simulink model "linear_feedback"  (R2021b)
settings: Solver=VariableStepAuto  StartTime=0.0  StopTime=10.0  RelTol=1e-3
undefined symbols (not defined in the file): magnitude
settings Model: Creator=84232  LastModifiedBy=84232

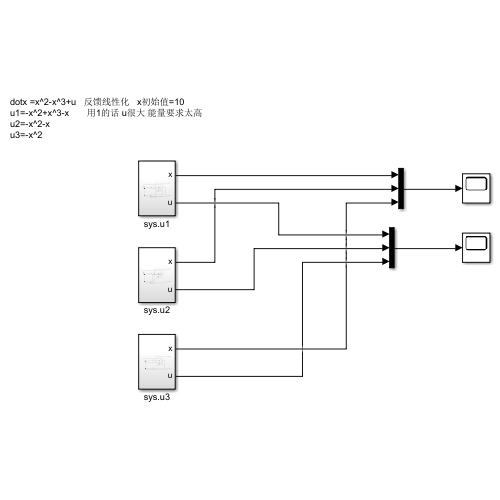
[thumbnail: Simulink's stored preview of the top-level diagram]
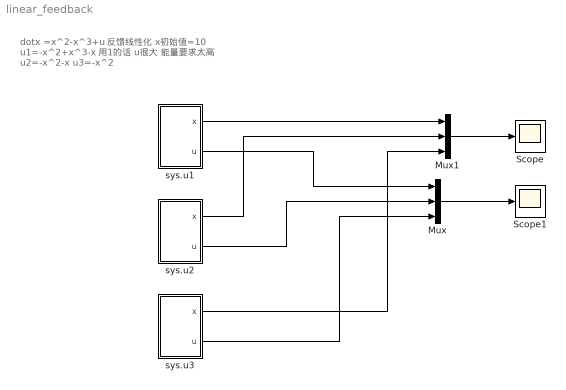
== system linear_feedback ==
  note: dotx =x^2-x^3+u   反馈线性化   x初始值=10
      | u1=-x^2+x^3-x       用1的话 u很大 能量要求太高
      | u2=-x^2-x
      | u3=-x^2
  Mux : Mux  Inputs=3
  Mux1 : Mux  Inputs=3
  Scope : Scope
  Scope1 : Scope
  sys.u1 : Subsystem
  sys.u2 : Subsystem
  sys.u3 : Subsystem
  wires:
  sys.u1/2(u) -> Mux/1
  sys.u2/2(u) -> Mux/2
  sys.u3/2(u) -> Mux/3
  Mux/1 -> Scope1/1
  sys.u1/1(x) -> Mux1/1
  sys.u2/1(x) -> Mux1/2
  sys.u3/1(x) -> Mux1/3
  Mux1/1 -> Scope/1

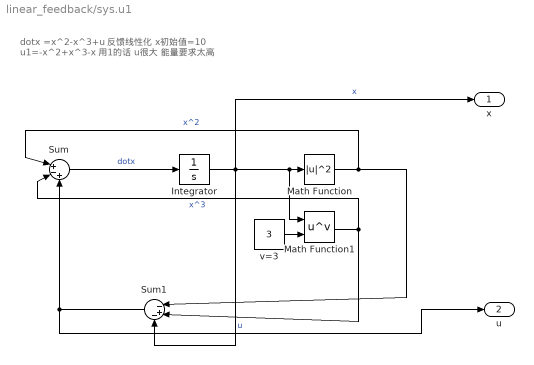
== system linear_feedback/sys.u1 ==
  note: dotx =x^2-x^3+u   反馈线性化   x初始值=10
      | u1=-x^2+x^3-x       用1的话 u很大 能量要求太高
  Integrator : Integrator  InitialCondition=10
  Math Function : Math  Operator=magnitude^2  SaturateOnIntegerOverflow=on
  Math Function1 : Math  Operator=pow  SaturateOnIntegerOverflow=on
  Sum : Sum  Inputs=|+-+
  Sum1 : Sum  Inputs=|-+-
  v=3 : Constant  Value=3
  x : Outport
  u : Outport  Port=2
  wires:
  Integrator/1 -> x/1, Sum1/3, Math Function1/1, Math Function/1  "x"
  Sum/1 -> Integrator/1  "dotx"
  v=3/1 -> Math Function1/2
  Math Function/1 -> Sum1/1, Sum/1  "x^2"
  Math Function1/1 -> Sum/2, Sum1/2  "x^3"
  Sum1/1 -> u/1, Sum/3  "u"

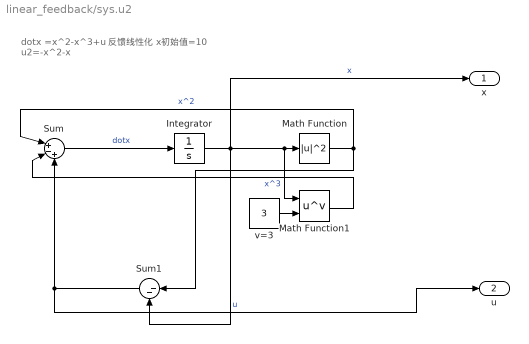
== system linear_feedback/sys.u2 ==
  note: dotx =x^2-x^3+u   反馈线性化   x初始值=10
      |
      | u2=-x^2-x
  Integrator : Integrator  InitialCondition=10
  Math Function : Math  Operator=magnitude^2  SaturateOnIntegerOverflow=on
  Math Function1 : Math  Operator=pow  SaturateOnIntegerOverflow=on
  Sum : Sum  Inputs=|+-+
  Sum1 : Sum  Inputs=|--
  v=3 : Constant  Value=3
  x : Outport
  u : Outport  Port=2
  wires:
  Integrator/1 -> Sum1/2, x/1, Math Function1/1, Math Function/1  "x"
  Sum/1 -> Integrator/1  "dotx"
  v=3/1 -> Math Function1/2
  Math Function/1 -> Sum1/1, Sum/1  "x^2"
  Math Function1/1 -> Sum/2  "x^3"
  Sum1/1 -> u/1, Sum/3  "u"

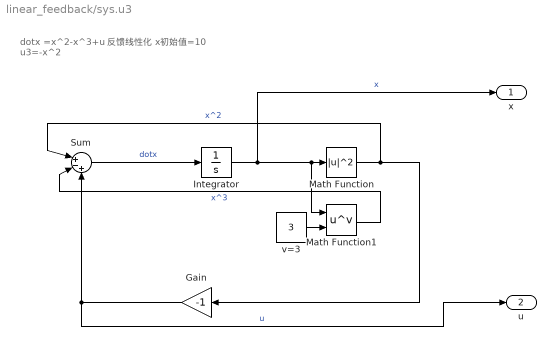
== system linear_feedback/sys.u3 ==
  note: dotx =x^2-x^3+u   反馈线性化   x初始值=10
      | u3=-x^2
  Gain : Gain  Gain=-1
  Integrator : Integrator  InitialCondition=10
  Math Function : Math  Operator=magnitude^2  SaturateOnIntegerOverflow=on
  Math Function1 : Math  Operator=pow  SaturateOnIntegerOverflow=on
  Sum : Sum  Inputs=|+-+
  v=3 : Constant  Value=3
  x : Outport
  u : Outport  Port=2
  wires:
  Integrator/1 -> x/1, Math Function1/1, Math Function/1  "x"
  Sum/1 -> Integrator/1  "dotx"
  v=3/1 -> Math Function1/2
  Math Function/1 -> Sum/1, Gain/1  "x^2"
  Math Function1/1 -> Sum/2  "x^3"
  Gain/1 -> u/1, Sum/3  "u"
